simulink model "Battery_pack"  (R2014a)
settings: Solver=ode23s  StartTime=0.0  StopTime=max(Idc.Time)  MaxStep=3  RelTol=1e-3
model workspace: external: MAT-File /Users/abk/Dropbox/Documents/OSU/Buckeye Current/Code/SimBALink/Model/Powertrain/Battery pack/Data/Raw/Battery pack.mat (data not in the file)
undefined symbols (not defined in the file or in its folder): C1, magnitude, Q_0, R0, R1, T_0, Vc0, Voc
settings Model: Creator=bonnella  LastModifiedBy=abk
settings DataIOCC: LimitDataPoints=off

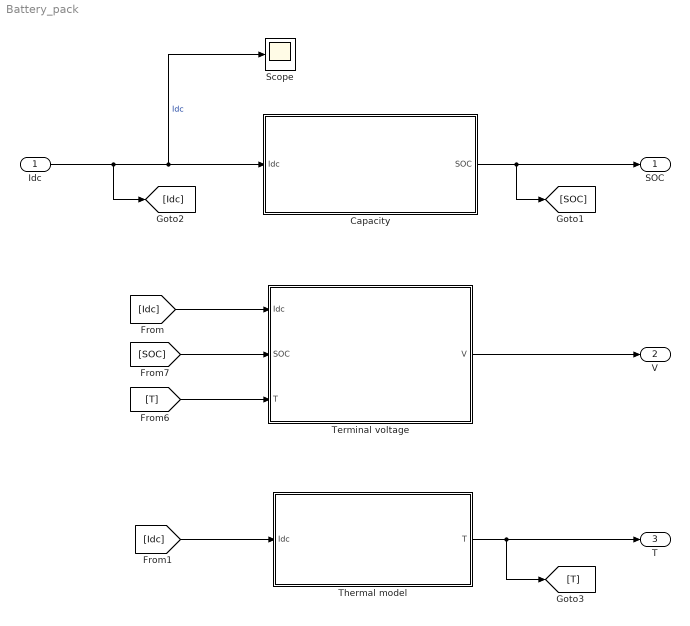
== system Battery_pack ==
  Idc : Inport
  Capacity : Subsystem
  Scope : Scope
  Terminal voltage : Subsystem
  Thermal model : Subsystem
  SOC : Outport
  V : Outport  Port=2
  T : Outport  Port=3
  wires:
  Terminal voltage/1(V) -> V/1
  [Idc] -> Terminal voltage/1(Idc)
  [SOC] -> Terminal voltage/2(SOC)
  [T] -> Terminal voltage/3(T)
  Idc/1 -> [Idc], Scope/1, Capacity/1(Idc)  "Idc"
  Capacity/1(SOC) -> [SOC], SOC/1
  [Idc] -> Thermal model/1(Idc)
  Thermal model/1(T) -> [T], T/1

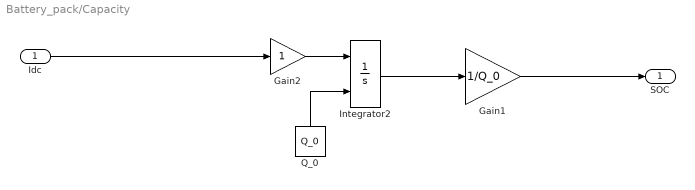
== system Battery_pack/Capacity ==
  Idc : Inport
  Gain1 : Gain  Gain=1/Q_0
  Gain2 : Gain
  Integrator2 : Integrator  InitialConditionSource=external  InitialCondition=Vc0
  Q_0 : Constant  Value=Q_0
  SOC : Outport
  wires:
  Q_0/1 -> Integrator2/2
  Gain2/1 -> Integrator2/1
  Integrator2/1 -> Gain1/1
  Idc/1 -> Gain2/1
  Gain1/1 -> SOC/1

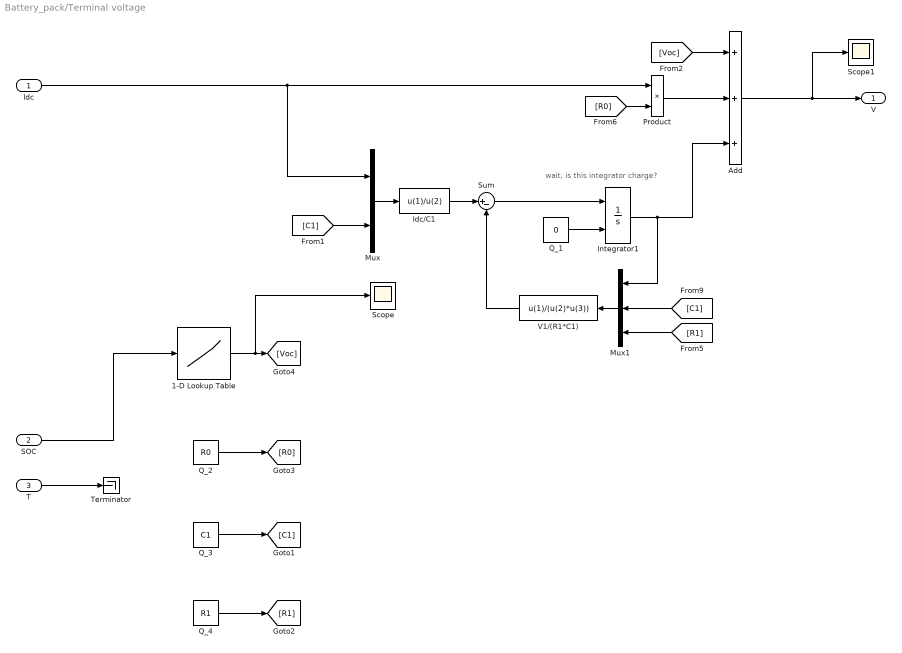
== system Battery_pack/Terminal voltage ==
  note: wait, is this integrator charge?
  Idc : Inport
  SOC : Inport  Port=2
  T : Inport  Port=3
  1-D Lookup Table : Lookup_n-D  NumberOfTableDimensions=1  BreakpointsForDimension1=Voc.SOC  Table=Voc.V  InternalRulePriority=Speed  RndMeth=Simplest  InputSameDT=on
  Add : Sum  Inputs=+++
  Idc/C1 : Fcn  Expr=u(1)/u(2)
  Integrator1 : Integrator  InitialConditionSource=external  InitialCondition=Vc0
  Mux : Mux  Inputs=2
  Mux1 : Mux  Inputs=3
  Product : Product  RndMeth=Zero
  Q_1 : Constant  Value=0
  Q_2 : Constant  Value=R0
  Q_3 : Constant  Value=C1
  Q_4 : Constant  Value=R1
  Scope : Scope
  Scope1 : Scope
      settings: YMin=3.5  YMax=8.5  SaveName=ScopeData2
  Sum : Sum  Inputs=|+-
  Terminator : Terminator
  V1/(R1*C1) : Fcn  Expr=u(1)/(u(2)*u(3))
  V : Outport
  wires:
  Q_3/1 -> [C1]
  Integrator1/1 -> Mux1/1, Add/3
  Product/1 -> Add/2
  [C1] -> Mux1/2
  Idc/1 -> Product/1, Mux/1
  Mux1/1 -> V1/(R1*C1)/1
  Mux/1 -> Idc/C1/1
  Add/1 -> Scope1/1, V/1
  Sum/1 -> Integrator1/1
  Idc/C1/1 -> Sum/1
  V1/(R1*C1)/1 -> Sum/2
  [R1] -> Mux1/3
  Q_4/1 -> [R1]
  [R0] -> Product/2
  SOC/1 -> 1-D Lookup Table/1
  Q_2/1 -> [R0]
  [C1] -> Mux/2
  [Voc] -> Add/1
  1-D Lookup Table/1 -> Scope/1, [Voc]
  T/1 -> Terminator/1
  Q_1/1 -> Integrator1/2

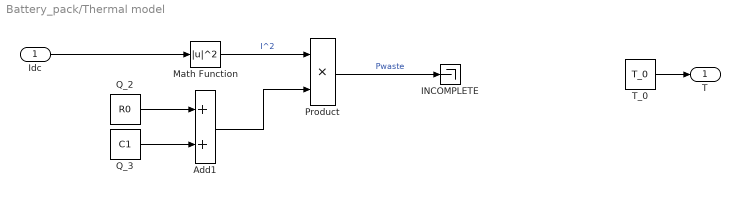
== system Battery_pack/Thermal model ==
  Idc : Inport
  Add1 : Sum
  INCOMPLETE : Terminator
  Math Function : Math  Operator=magnitude^2  SaturateOnIntegerOverflow=on
  Product : Product  RndMeth=Zero
  Q_2 : Constant  Value=R0
  Q_3 : Constant  Value=C1
  T_0 : Constant  Value=T_0
  T : Outport
  wires:
  Q_3/1 -> Add1/2
  Idc/1 -> Math Function/1
  Q_2/1 -> Add1/1
  Math Function/1 -> Product/1  "I^2"
  Add1/1 -> Product/2
  Product/1 -> INCOMPLETE/1  "Pwaste"
  T_0/1 -> T/1
